simulink subsystem "SF_MetricsEvaluation"  (R2022b)
settings: Solver=VariableStepAuto  StartTime=0.0  StopTime=10.0  RelTol=1e-3
settings Model: Creator=smryk  LastModifiedBy=smryk

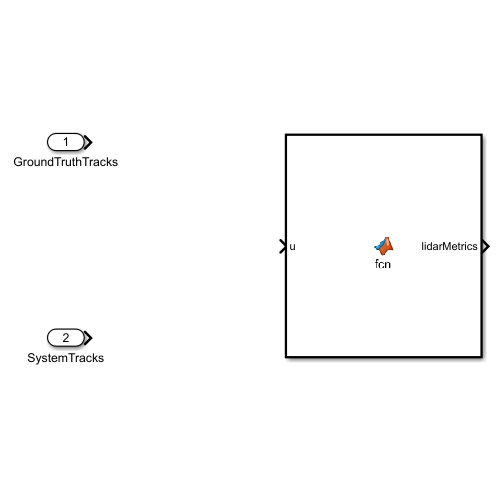
[thumbnail: Simulink's stored preview of the top-level diagram]
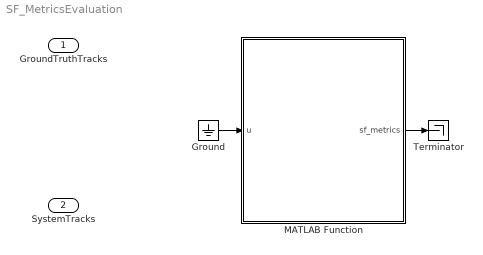
== system SF_MetricsEvaluation ==
  GroundTruthTracks : Inport  OutDataTypeStr=Bus: BusActors1
  SystemTracks : Inport  Port=2  OutDataTypeStr=Bus: SystemTracks
  Ground : Ground
  MATLAB Function : MATLAB Function  TreatAsAtomicUnit=on
  Terminator : Terminator
  wires:
  Ground/1 -> MATLAB Function/1(u)
  MATLAB Function/1(sf_metrics) -> Terminator/1

== matlab function SF_MetricsEvaluation/MATLAB Function ==
  data: u input; sf_metrics output
function sf_metrics = fcn(u)

sf_metrics = u;
